simulink model "sampleModel84"  (Simulink 9.1)
settings: Solver=VariableStepAuto  StartTime=0.0  StopTime=10.0  RelTol=1e-3
undefined symbols (not defined in the file): DiscIntNeverNeededParam, Newton, Raphson
libraries: simulink x55
(part 1 of 2)
settings Model: SuppressorTable="22 serialization::archive 11 0 6 0 0 1 8 0 0 0 0 6 0 0 1 0 21 sampleModel84/cfblk80 0 6 0 0 2 8 0 0 0 0 6 41 Simulink:DataType:WarningOverFlowDetected 0 0 0 6 0  0  0 0 0 0 8 20160523 0 0 0 10 57 55 0 1 40 SimulinkFixedPoint:util:Overflowoccurred 0 0 0  0  8 20160523 0 10 57 55 0 1"  Creator=DELL  LastModifiedBy=DELL
settings DataIOCC: SaveFormat=Dataset
settings OptimizationCC: LifeSpan=auto
settings DebuggingCC: UnderspecifiedInitializationDetection=Simplified  MergeDetectMultiDrivingBlocksExec=error  SFUnexpectedBacktrackingDiag=error  SFNoUnconditionalDefaultTransitionDiag=error  SFExecutionAtInitializationDiag=warning
settings HardwareCC: ProdBitPerPointer=64  ProdBitPerSizeT=64  ProdBitPerPtrDiffT=64  ProdLargestAtomicFloat=Float  ProdIntDivRoundTo=Zero  ProdEndianess=LittleEndian  ProdWordSize=64  ProdHWDeviceType=Intel->x86-64 (Windows64)
settings ModelReferenceCC: PropagateSignalLabelsOutOfModel=on
settings CodeAppCC: StateflowObjectComments=off
settings GRTTargetCC: TargetLangStandard=C99 (ISO)  CombineOutputUpdateFcns=on  GRTInterface=off
settings ConfigComp: CovMetricSettings=dwe  CovHtmlReporting=off  CovSaveCumulativeToWorkspaceVar=off  CovSaveSingleToWorkspaceVar=off  CovExternalEMLEnable=on

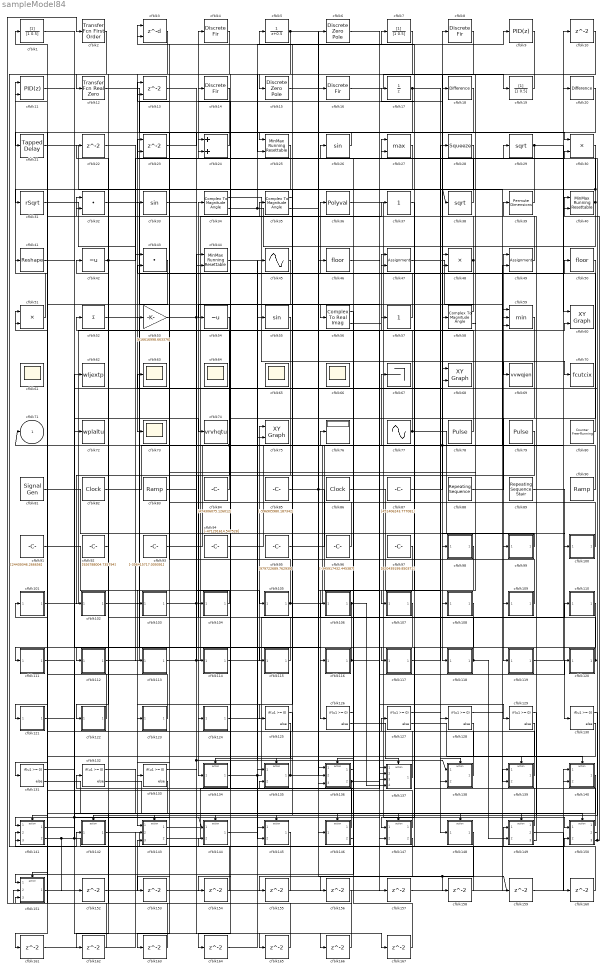
== system sampleModel84 ==
  cfblk1 : DiscreteFilter  SampleTime=1
  cfblk{10,22,152..167} (18 alike) : Delay  SampleTime=1
  cfblk100 : Subsystem
  cfblk101 : Subsystem
  cfblk102 : Subsystem
  cfblk103 : Subsystem
  cfblk104 : Subsystem
  cfblk105 : Subsystem
  cfblk106 : Subsystem
  cfblk107 : Subsystem
  cfblk108 : Subsystem
  cfblk109 : Subsystem
  cfblk11 : simulink/Continuous/PID Controller (2DOF)  Controller=PID  TimeDomain=Discrete-time  SampleTime=1  IntegratorMethod=Forward Euler  FilterMethod=Forward Euler  Form=Parallel  UseFilter=on  ControllerParametersSource=internal  P=1  I=1  D=0  N=100  b=1  c=1  InitialConditionSource=internal  InitialConditionForIntegrator=0  InitialConditionForFilter=0  ExternalReset=none  LimitOutput=off  UpperSaturationLimit=inf  LowerSaturationLimit=-inf  LinearizeAsGain=off  AntiWindupMode=none  Kb=1  TrackingMode=off  Kt=1  PParamMin=[]  PParamMax=[]  IParamMin=[]  IParamMax=[]  DParamMin=[]  DParamMax=[]  NParamMin=[]  NParamMax=[]  bParamMin=[]  bParamMax=[]  cParamMin=[]  cParamMax=[]  KbParamMin=[]  KbParamMax=[]  KtParamMin=[]  KtParamMax=[]  POutMin=[]  POutMax=[]  IOutMin=[]  IOutMax=[]  DOutMin=[]  DOutMax=[]  NOutMin=[]  NOutMax=[]  bOutMin=[]  bOutMax=[]  cOutMin=[]  cOutMax=[]  KbOutMin=[]  KbOutMax=[]  KtOutMin=[]  KtOutMax=[]  IntegratorOutMin=[]  IntegratorOutMax=[]  FilterOutMin=[]  FilterOutMax=[]  SumOutMin=[]  SumOutMax=[]  Sum1OutMin=[]  Sum1OutMax=[]  Sum2OutMin=[]  Sum2OutMax=[]  Sum3OutMin=[]  Sum3OutMax=[]  SumI1OutMin=[]  SumI1OutMax=[]  SumI2OutMin=[]  SumI2OutMax=[]  SumI3OutMin=[]  SumI3OutMax=[]  SumDOutMin=[]  SumDOutMax=[]  SaturationOutMin=[]  SaturationOutMax=[]  IntegratorContinuousStateAttributes=''  IntegratorStateMustResolveToSignalObject=off  IntegratorRTWStateStorageClass=Auto  FilterContinuousStateAttributes=''  FilterStateMustResolveToSignalObject=off  FilterRTWStateStorageClass=Auto  DifferentiatorICPrevScaledInput=0  DifferentiatorOutMin=[]  DifferentiatorOutMax=[]  FilterDiffOutCoefMin=[]  FilterDiffOutCoefMax=[]  SumDenOutMin=[]  SumDenOutMax=[]  SumNumOutMin=[]  SumNumOutMax=[]  ReciprocalOutMin=[]  ReciprocalOutMax=[]  DivideOutMin=[]  DivideOutMax=[]  TunerSelectOption=Transfer Function Based (PID Tuner App)
  cfblk110 : Subsystem
  cfblk111 : Subsystem
  cfblk112 : Subsystem
  cfblk113 : Subsystem
  cfblk114 : Subsystem
  cfblk115 : Subsystem
  cfblk116 : Subsystem
  cfblk117 : Subsystem
  cfblk118 : Subsystem
  cfblk119 : Subsystem
  cfblk12 : simulink/Discrete/Transfer Fcn Real Zero  ZeroZ=0.75  ICPrevInput=0.0  DoSatur=off
      settings: SourceProductName=Simulink  SourceProductBaseCode=SL
  cfblk120 : Subsystem
  cfblk121 : Subsystem
  cfblk122 : Subsystem
  cfblk123 : Subsystem
  cfblk124 : Subsystem
  cfblk{125..133} (9 alike) : If  IfExpression=u1 >= 0  SampleTime=1
  cfblk13 : Delay  ShowEnablePort=on  SampleTime=1
      settings: InputPortMap=u0,e6
  cfblk134 : Subsystem  TreatAsAtomicUnit=on
  cfblk135 : Subsystem  TreatAsAtomicUnit=on
  cfblk136 : Subsystem  TreatAsAtomicUnit=on
  cfblk137 : Subsystem  TreatAsAtomicUnit=on
  cfblk138 : Subsystem  TreatAsAtomicUnit=on
  cfblk139 : Subsystem  TreatAsAtomicUnit=on
  cfblk{4,8,14,16} (4 alike) : DiscreteFir  SampleTime=1
  cfblk140 : Subsystem  TreatAsAtomicUnit=on
  cfblk141 : Subsystem  TreatAsAtomicUnit=on
  cfblk142 : Subsystem  TreatAsAtomicUnit=on
  cfblk143 : Subsystem  TreatAsAtomicUnit=on
  cfblk144 : Subsystem  TreatAsAtomicUnit=on
  cfblk145 : Subsystem  TreatAsAtomicUnit=on
  cfblk146 : Subsystem  TreatAsAtomicUnit=on
  cfblk147 : Subsystem  TreatAsAtomicUnit=on
  cfblk148 : Subsystem  TreatAsAtomicUnit=on
  cfblk149 : Subsystem  TreatAsAtomicUnit=on
  cfblk15 : DiscreteZeroPole  Poles=[0 0.5]  Gain=1
  cfblk150 : Subsystem  TreatAsAtomicUnit=on
  cfblk151 : Subsystem  TreatAsAtomicUnit=on
  cfblk17 : UnitDelay
  cfblk18 : simulink/Discrete/Difference  ICPrevInput=0.0  OutMin=[]  OutMax=[]  OutDataTypeStr=Inherit: Inherit via back propagation  OutDataType=fixdt(1, 16)  OutScaling=2^-10  DoSatur=off
  cfblk19 : DiscreteFilter  SampleTime=1
  cfblk2 : simulink/Discrete/Transfer Fcn First Order  PoleZ=0.95  ICPrevOutput=0.0  DoSatur=off
      settings: SourceProductName=Simulink
  cfblk20 : simulink/Discrete/Difference  ICPrevInput=0.0  OutMin=[]  OutMax=[]  OutDataTypeStr=Inherit: Inherit via back propagation  OutDataType=fixdt(1, 16)  OutScaling=2^-10  DoSatur=off
  cfblk21 : simulink/Discrete/Tapped Delay  vinit=0.0  samptime=-1  NumDelays=1  DelayOrder=Oldest  includeCurrent=off
  cfblk23 : Delay  ShowEnablePort=on  SampleTime=1
      settings: InputPortMap=u0,e6
  cfblk24 : Sum
  cfblk25 : simulink/Math Operations/MinMax Running Resettable  Function=min  vinit=0.0
  cfblk26 : Trigonometry
  cfblk27 : MinMax  Function=max  Inputs=2
  cfblk28 : Squeeze
  cfblk29 : Sqrt  SaturateOnIntegerOverflow=on
  cfblk3 : Delay  DelayLengthSource=Input port  SampleTime=1
      settings: InputPortMap=u0,p1
  cfblk30 : Product
  cfblk31 : Sqrt  Operator=rSqrt  AlgorithmType=Newton-Raphson  SaturateOnIntegerOverflow=on
  cfblk32 : DotProduct  InputSameDT=on  OutDataTypeStr=Inherit: Inherit via internal rule
  cfblk33 : Trigonometry
  cfblk34 : ComplexToMagnitudeAngle
  cfblk35 : ComplexToMagnitudeAngle
  cfblk36 : Polyval  Coefs=[ +2.081618890e-019, -1.441693666e-014, +4.719686976e-010, -8.536869453e-006, +1.621573104e-001, -8.087801117e+001 ]
  cfblk37 : simulink/Math Operations/Slider Gain  gain=1  low=0  high=2
  cfblk38 : Sqrt  SaturateOnIntegerOverflow=on
  cfblk39 : PermuteDimensions
  cfblk40 : simulink/Math Operations/MinMax Running Resettable  Function=min  vinit=0.0
  cfblk41 : Reshape
  cfblk42 : UnaryMinus
  cfblk43 : DotProduct  InputSameDT=on  OutDataTypeStr=Inherit: Inherit via internal rule
  cfblk44 : simulink/Math Operations/MinMax Running Resettable  Function=min  vinit=0.0
  cfblk45 : Sin  TimeSource=Use external signal  SampleTime=0
  cfblk46 : Rounding
  cfblk47 : Assignment  DiagnosticForDimensions=Warning  IndexOptions=Index vector (dialog)  Indices=1  OutputSizes=1
  cfblk48 : Product  Inputs=**
  cfblk49 : Assignment  DiagnosticForDimensions=Warning  IndexOptions=Index vector (dialog)  Indices=1  OutputSizes=1
  cfblk5 : DiscreteTransferFcn  SampleTime=1
  cfblk50 : Rounding
  cfblk51 : Product  Inputs=**
  cfblk52 : Sum  Inputs=+
  cfblk53 : Gain  Gain=[616616998.663376]
  cfblk54 : UnaryMinus
  cfblk55 : Trigonometry
  cfblk56 : ComplexToRealImag
  cfblk57 : simulink/Math Operations/Slider Gain  gain=1  low=0  high=2
  cfblk58 : ComplexToMagnitudeAngle
  cfblk59 : MinMax  Inputs=3
  cfblk6 : DiscreteZeroPole  Poles=[0 0.5]  Gain=1
  cfblk60 : simulink/Sinks/XY Graph  xmin=-1  xmax=1  ymin=-1  ymax=1  st=-1
  cfblk{61,63..66,73} (6 alike) : Scope
      cfblk61 settings: Floating=on
      cfblk64 settings: Floating=on
      cfblk65 settings: Floating=on
      cfblk66 settings: Floating=on
  cfblk62 : ToWorkspace  VariableName=wljextp  SaveFormat=Timeseries  SampleTime=-1
  cfblk67 : Terminator
  cfblk68 : simulink/Sinks/XY Graph  xmin=-1  xmax=1  ymin=-1  ymax=1  st=-1
  cfblk69 : ToWorkspace  VariableName=vvwqjen  SaveFormat=Timeseries  SampleTime=-1
  cfblk7 : DiscreteFilter  SampleTime=1
  cfblk70 : ToWorkspace  VariableName=fcutcix  SaveFormat=Timeseries  SampleTime=-1
  cfblk72 : ToWorkspace  VariableName=wplaltu  SaveFormat=Timeseries  SampleTime=-1
  cfblk74 : ToWorkspace  VariableName=vrvhqtu  SaveFormat=Timeseries  SampleTime=-1
  cfblk75 : simulink/Sinks/XY Graph  xmin=-1  xmax=1  ymin=-1  ymax=1  st=-1
  cfblk76 : Display
  cfblk77 : Sin  Amplitude=[108722307.929304]  Bias=[-485802792.606317]  SampleTime=0
  cfblk78 : DiscretePulseGenerator  PulseType=Time based  Amplitude=[385040075.509657]  Period=[73350272.641050]  PulseWidth=5  PhaseDelay=[8.000000]
  cfblk79 : DiscretePulseGenerator  PulseType=Time based  Amplitude=[-502906939.049966]  Period=[87047927.574360]  PulseWidth=5  PhaseDelay=[5.000000]
  cfblk80 : simulink/Sources/Counter Free-Running  NumBits=[10.000000]  tsamp=-1
  cfblk81 : SignalGenerator  WaveForm=sawtooth  Amplitude=[-168191478.001369]  Units=rad/sec
  cfblk82 : DigitalClock
  cfblk83 : simulink/Sources/Ramp  slope=[-4630.726628]  start=[27.607635]  InitialOutput=[-903636.017661]
  cfblk84 : Constant  Value=[474306075.126012]  SampleTime=1
  cfblk85 : Constant  Value=[-596905980.187342]  SampleTime=1
  cfblk86 : DigitalClock
  cfblk87 : Constant  Value=[451406243.777081]  SampleTime=1
  cfblk88 : simulink/Sources/Repeating Sequence  rep_seq_t=[0 2]  rep_seq_y=[-211485447.920603, -631862851.400654]
  cfblk89 : simulink/Sources/Repeating Sequence Stair  OutValues=[504633055.748347, -907869422.671242]  tsamp=-1  OutMin=[]  OutMax=[]  OutDataTypeStr=double  OutputDataTypeScalingMode=double  OutDataType=fixdt(0,8)  ConRadixGroup=Best Precision: Vector-wise  OutScaling=2^-12
  cfblk9 : simulink/Continuous/PID Controller  Controller=PID  TimeDomain=Discrete-time  SampleTime=1  IntegratorMethod=Forward Euler  FilterMethod=Forward Euler  Form=Parallel  UseFilter=on  ControllerParametersSource=internal  P=1  I=1  D=0  N=100  InitialConditionSource=internal  InitialConditionForIntegrator=0  InitialConditionForFilter=0  ExternalReset=none  LimitOutput=off  UpperSaturationLimit=inf  LowerSaturationLimit=-inf  LinearizeAsGain=off  AntiWindupMode=none  Kb=1  TrackingMode=off  Kt=1  PParamMin=[]  PParamMax=[]  IParamMin=[]  IParamMax=[]  DParamMin=[]  DParamMax=[]  NParamMin=[]  NParamMax=[]  KbParamMin=[]  KbParamMax=[]  KtParamMin=[]  KtParamMax=[]  POutMin=[]  POutMax=[]  IOutMin=[]  IOutMax=[]  DOutMin=[]  DOutMax=[]  NOutMin=[]  NOutMax=[]  KbOutMin=[]  KbOutMax=[]  KtOutMin=[]  KtOutMax=[]  IntegratorOutMin=[]  IntegratorOutMax=[]  FilterOutMin=[]  FilterOutMax=[]  SumOutMin=[]  SumOutMax=[]  SumI1OutMin=[]  SumI1OutMax=[]  SumI2OutMin=[]  SumI2OutMax=[]  SumI3OutMin=[]  SumI3OutMax=[]  SumDOutMin=[]  SumDOutMax=[]  SaturationOutMin=[]  SaturationOutMax=[]  IntegratorContinuousStateAttributes=''  IntegratorStateMustResolveToSignalObject=off  IntegratorRTWStateStorageClass=Auto  FilterContinuousStateAttributes=''  FilterStateMustResolveToSignalObject=off  FilterRTWStateStorageClass=Auto  DifferentiatorICPrevScaledInput=0  DifferentiatorOutMin=[]  DifferentiatorOutMax=[]  FilterDiffOutCoefMin=[]  FilterDiffOutCoefMax=[]  SumDenOutMin=[]  SumDenOutMax=[]  SumNumOutMin=[]  SumNumOutMax=[]  ReciprocalOutMin=[]  ReciprocalOutMax=[]  DivideOutMin=[]  DivideOutMax=[]  TunerSelectOption=Transfer Function Based (PID Tuner App)
  cfblk90 : simulink/Sources/Ramp  slope=[-8360.756305]  start=[2.779328]  InitialOutput=[-108037.496599]
  cfblk91 : Constant  Value=[24439346.266656]  SampleTime=1
  cfblk92 : Constant  Value=[926788004.735794]  SampleTime=1
  cfblk93 : Constant  Value=[-356415717.009391]  SampleTime=1
  cfblk94 : Constant  Value=[-471291614.547528]  SampleTime=1
  cfblk95 : Constant  Value=[979722689.762939]  SampleTime=1
  cfblk96 : Constant  Value=[-345917432.445387]  SampleTime=1
  cfblk97 : Constant  Value=[820439199.850371]  SampleTime=1
  cfblk98 : Subsystem
  cfblk99 : Subsystem
  cfblk71 : Outport
  wires:
  cfblk82/1 -> cfblk8/1
  cfblk79/1 -> cfblk134/1(cfblk1)
  cfblk57/1 -> cfblk36/1
  cfblk97/1 -> cfblk126/1
  cfblk9/1 -> cfblk141/1(cfblk1)
  cfblk116/1(cfblk2) -> cfblk111/1(cfblk1), cfblk129/1
  cfblk52/1 -> cfblk116/1(cfblk1)
  cfblk2/1 -> cfblk142/1(cfblk1)
  cfblk89/1 -> cfblk130/1
  cfblk56/1 -> cfblk151/1(cfblk1)
  cfblk91/1 -> cfblk143/1(cfblk1)
  cfblk51/1 -> cfblk11/1
  cfblk84/1 -> cfblk71/1, cfblk13/2
  cfblk36/1 -> cfblk150/1(cfblk1)
  cfblk106/1(cfblk2) -> cfblk121/1(cfblk1), cfblk137/4(cfblk9)
  cfblk102/1(cfblk2) -> cfblk50/1
  cfblk8/1 -> cfblk118/1(cfblk1)
  cfblk93/1 -> cfblk48/1
  cfblk87/1 -> cfblk58/1
  cfblk137/1(cfblk2) -> cfblk26/1
  cfblk101/1(cfblk2) -> cfblk47/1
  cfblk113/1(cfblk2) -> cfblk37/1, cfblk48/2
  cfblk3/1 -> cfblk112/1(cfblk1)
  cfblk81/1 -> cfblk100/1(cfblk1)
  cfblk59/1 -> cfblk119/1(cfblk1)
  cfblk77/1 -> cfblk109/1(cfblk1), cfblk32/2
  cfblk37/1 -> cfblk107/1(cfblk1)
  cfblk5/1 -> cfblk158/1, cfblk159/1, cfblk25/2
  cfblk56/2 -> cfblk57/1
  cfblk112/1(cfblk2) -> cfblk18/1
  cfblk34/1 -> cfblk70/1
  cfblk119/1(cfblk2) -> cfblk20/1
  cfblk90/1 -> cfblk42/1, cfblk68/1
  cfblk35/1 -> cfblk123/1(cfblk1)
  cfblk40/1 -> cfblk38/1, cfblk13/1, cfblk138/2(cfblk11)
  cfblk136/1(cfblk2) -> cfblk76/1
  cfblk95/1 -> cfblk67/1
  cfblk118/1(cfblk2) -> cfblk34/1, cfblk149/2(cfblk13)
  cfblk7/1 -> cfblk54/1
  cfblk10/1 -> cfblk12/1
  cfblk14/1 -> cfblk73/1
  cfblk142/1(cfblk2) -> cfblk150/2(cfblk8)
  cfblk88/1 -> cfblk49/1
  cfblk38/1 -> cfblk4/1
  cfblk45/1 -> cfblk114/1(cfblk1)
  cfblk17/1 -> cfblk99/1(cfblk1), cfblk163/1
  cfblk114/1(cfblk2) -> cfblk75/1
  cfblk16/1 -> cfblk19/1
  cfblk99/1(cfblk2) -> cfblk98/1(cfblk1)
  cfblk151/1(cfblk2) -> cfblk55/1
  cfblk78/1 -> cfblk24/1
  cfblk149/1(cfblk2) -> cfblk3/1
  cfblk141/1(cfblk2) -> cfblk62/1
  cfblk47/1 -> cfblk139/2(cfblk12)
  cfblk4/1 -> cfblk53/1
  cfblk1/1 -> cfblk74/1
  cfblk20/1 -> cfblk131/1
  cfblk146/1(cfblk2) -> cfblk14/1
  cfblk33/1 -> cfblk105/1(cfblk1)
  cfblk96/1 -> cfblk23/1
  cfblk28/1 -> cfblk31/1
  cfblk48/1 -> cfblk1/1, cfblk75/2
  cfblk32/1 -> cfblk137/1(cfblk1)
  cfblk134/1(cfblk2) -> cfblk6/1, cfblk147/2(cfblk6)
  cfblk109/1(cfblk2) -> cfblk35/1
  cfblk124/1(cfblk2) -> cfblk16/1
  cfblk139/1(cfblk2) -> cfblk24/2
  cfblk100/1(cfblk2) -> cfblk23/2
  cfblk22/1 -> cfblk43/1
  cfblk108/1(cfblk2) -> cfblk117/1(cfblk1)
  cfblk86/1 -> cfblk128/1
  cfblk12/1 -> cfblk146/1(cfblk1)
  cfblk145/1(cfblk2) -> cfblk141/2(cfblk15)
  cfblk115/1(cfblk2) -> cfblk32/1
  cfblk31/1 -> cfblk113/1(cfblk1)
  cfblk85/1 -> cfblk136/1(cfblk1), cfblk137/3(cfblk8)
  cfblk35/2 -> cfblk27/1
  cfblk53/1 -> cfblk138/1(cfblk1), cfblk165/1, cfblk47/2
  cfblk42/1 -> cfblk122/1(cfblk1), cfblk30/2
  cfblk54/1 -> cfblk104/1(cfblk1)
  cfblk80/1 -> cfblk3/2
  cfblk39/1 -> cfblk33/1
  cfblk107/1(cfblk2) -> cfblk133/1
  cfblk11/1 -> cfblk115/1(cfblk1)
  cfblk120/1(cfblk2) -> cfblk27/2, cfblk40/2
  cfblk30/1 -> cfblk125/1
  cfblk150/1(cfblk2) -> cfblk7/1
  cfblk135/1(cfblk2) -> cfblk110/1(cfblk1), cfblk101/1(cfblk1)
  cfblk26/1 -> cfblk25/1
  cfblk58/1 -> cfblk56/1
  cfblk24/1 -> cfblk21/1
  cfblk150/2(cfblk9) -> cfblk63/1
  cfblk83/1 -> cfblk44/1
  cfblk21/1 -> cfblk59/1
  cfblk92/1 -> cfblk22/1
  cfblk143/1(cfblk2) -> cfblk135/2(cfblk10)
  cfblk123/1(cfblk2) -> cfblk51/1
  cfblk18/1 -> cfblk124/1(cfblk1)
  cfblk144/1(cfblk2) -> cfblk45/1
  cfblk141/2(cfblk17) -> cfblk149/1(cfblk1), cfblk68/2, cfblk152/1
  cfblk13/1 -> cfblk137/2(cfblk7)
  cfblk41/1 -> cfblk72/1
  cfblk149/3(cfblk15) -> cfblk39/1
  cfblk29/1 -> cfblk60/1, cfblk59/3
  cfblk55/1 -> cfblk102/1(cfblk1)
  cfblk105/1(cfblk2) -> cfblk43/2, cfblk49/2
  cfblk44/1 -> cfblk136/2(cfblk11)
  cfblk150/3(cfblk10) -> cfblk40/1, cfblk29/1
  cfblk103/1(cfblk2) -> cfblk145/2(cfblk10), cfblk59/2
  cfblk6/1 -> cfblk69/1
  cfblk94/1 -> cfblk10/1
  cfblk146/2(cfblk16) -> cfblk132/1
  cfblk19/1 -> cfblk15/1
  cfblk143/2(cfblk17) -> cfblk120/1(cfblk1)
  cfblk122/1(cfblk2) -> cfblk41/1
  cfblk34/2 -> cfblk148/1(cfblk1), cfblk9/1
  cfblk110/1(cfblk2) -> cfblk147/1(cfblk1)
  cfblk117/1(cfblk2) -> cfblk28/1
  cfblk58/2 -> cfblk108/1(cfblk1)
  cfblk98/1(cfblk2) -> cfblk136/3(cfblk12)
  cfblk27/1 -> cfblk44/2
  cfblk121/1(cfblk2) -> cfblk144/1(cfblk1), cfblk167/1
  cfblk147/1(cfblk2) -> cfblk51/2
  cfblk49/1 -> cfblk17/1
  cfblk23/1 -> cfblk30/1
  cfblk15/1 -> cfblk46/1
  cfblk104/1(cfblk2) -> cfblk103/1(cfblk1)
  cfblk136/2(cfblk13) -> cfblk60/2, cfblk162/1
  cfblk138/1(cfblk2) -> cfblk5/1
  cfblk125/1 -> cfblk134/Action
  cfblk125/2 -> cfblk135/Action
  cfblk126/1 -> cfblk136/Action
  cfblk126/2 -> cfblk137/Action
  cfblk127/1 -> cfblk138/Action
  cfblk127/2 -> cfblk139/Action
  cfblk128/1 -> cfblk140/Action
  cfblk128/2 -> cfblk141/Action
  cfblk129/1 -> cfblk142/Action
  cfblk129/2 -> cfblk143/Action
  cfblk130/1 -> cfblk144/Action
  cfblk130/2 -> cfblk145/Action
  cfblk131/1 -> cfblk146/Action
  cfblk131/2 -> cfblk147/Action
  cfblk132/1 -> cfblk148/Action
  cfblk132/2 -> cfblk149/Action
  cfblk133/1 -> cfblk150/Action
  cfblk133/2 -> cfblk151/Action
  cfblk152/1 -> cfblk143/3(cfblk16)
  cfblk25/1 -> cfblk153/1
  cfblk153/1 -> cfblk140/1(cfblk1)
  cfblk140/1(cfblk2) -> cfblk154/1
  cfblk154/1 -> cfblk11/2
  cfblk147/2(cfblk7) -> cfblk155/1
  cfblk155/1 -> cfblk144/2(cfblk17)
  cfblk148/1(cfblk2) -> cfblk156/1
  cfblk156/1 -> cfblk2/1
  cfblk46/1 -> cfblk157/1
  cfblk157/1 -> cfblk139/1(cfblk1)
  cfblk158/1 -> cfblk145/1(cfblk1)
  cfblk159/1 -> cfblk140/2(cfblk15)
  cfblk149/2(cfblk14) -> cfblk160/1
  cfblk160/1 -> cfblk127/1
  cfblk43/1 -> cfblk161/1
  cfblk161/1 -> cfblk143/2(cfblk15)
  cfblk162/1 -> cfblk141/3(cfblk16)
  cfblk163/1 -> cfblk151/2(cfblk8)
  cfblk50/1 -> cfblk164/1
  cfblk164/1 -> cfblk135/1(cfblk1)
  cfblk165/1 -> cfblk151/3(cfblk9)
  cfblk111/1(cfblk2) -> cfblk166/1
  cfblk166/1 -> cfblk52/1
  cfblk167/1 -> cfblk106/1(cfblk1)

== system sampleModel84/cfblk100 ==
  cfblk1 : Inport
  cfblk2 : Outport
  wires:
  cfblk1/1 -> cfblk2/1

== system sampleModel84/cfblk101 ==
  cfblk1 : Inport
  cfblk2 : Outport
  wires:
  cfblk1/1 -> cfblk2/1

== system sampleModel84/cfblk102 ==
  cfblk1 : Inport
  cfblk2 : Outport
  wires:
  cfblk1/1 -> cfblk2/1

== system sampleModel84/cfblk103 ==
  cfblk1 : Inport
  cfblk2 : Outport
  wires:
  cfblk1/1 -> cfblk2/1

== system sampleModel84/cfblk104 ==
  cfblk1 : Inport
  cfblk2 : Outport
  wires:
  cfblk1/1 -> cfblk2/1

== system sampleModel84/cfblk105 ==
  cfblk1 : Inport
  cfblk2 : Outport
  wires:
  cfblk1/1 -> cfblk2/1

== system sampleModel84/cfblk106 ==
  cfblk1 : Inport
  cfblk2 : Outport
  wires:
  cfblk1/1 -> cfblk2/1

== system sampleModel84/cfblk107 ==
  cfblk1 : Inport
  cfblk2 : Outport
  wires:
  cfblk1/1 -> cfblk2/1

== system sampleModel84/cfblk108 ==
  cfblk1 : Inport
  cfblk2 : Outport
  wires:
  cfblk1/1 -> cfblk2/1

== system sampleModel84/cfblk109 ==
  cfblk1 : Inport
  cfblk2 : Outport
  wires:
  cfblk1/1 -> cfblk2/1

== system sampleModel84/cfblk110 ==
  cfblk1 : Inport
  cfblk2 : Outport
  wires:
  cfblk1/1 -> cfblk2/1

== system sampleModel84/cfblk111 ==
  cfblk1 : Inport
  cfblk2 : Outport
  wires:
  cfblk1/1 -> cfblk2/1

== system sampleModel84/cfblk112 ==
  cfblk1 : Inport
  cfblk2 : Outport
  wires:
  cfblk1/1 -> cfblk2/1

== system sampleModel84/cfblk113 ==
  cfblk1 : Inport
  cfblk2 : Outport
  wires:
  cfblk1/1 -> cfblk2/1

== system sampleModel84/cfblk114 ==
  cfblk1 : Inport
  cfblk2 : Outport
  wires:
  cfblk1/1 -> cfblk2/1

== system sampleModel84/cfblk115 ==
  cfblk1 : Inport
  cfblk2 : Outport
  wires:
  cfblk1/1 -> cfblk2/1

== system sampleModel84/cfblk116 ==
  cfblk1 : Inport
  cfblk2 : Outport
  wires:
  cfblk1/1 -> cfblk2/1

== system sampleModel84/cfblk117 ==
  cfblk1 : Inport
  cfblk2 : Outport
  wires:
  cfblk1/1 -> cfblk2/1

== system sampleModel84/cfblk118 ==
  cfblk1 : Inport
  cfblk2 : Outport
  wires:
  cfblk1/1 -> cfblk2/1

== system sampleModel84/cfblk119 ==
  cfblk1 : Inport
  cfblk2 : Outport
  wires:
  cfblk1/1 -> cfblk2/1

== system sampleModel84/cfblk120 ==
  cfblk1 : Inport
  cfblk2 : Outport
  wires:
  cfblk1/1 -> cfblk2/1

== system sampleModel84/cfblk121 ==
  cfblk1 : Inport
  cfblk2 : Outport
  wires:
  cfblk1/1 -> cfblk2/1

== system sampleModel84/cfblk122 ==
  cfblk1 : Inport
  cfblk2 : Outport
  wires:
  cfblk1/1 -> cfblk2/1

== system sampleModel84/cfblk123 ==
  cfblk1 : Inport
  cfblk2 : Outport
  wires:
  cfblk1/1 -> cfblk2/1

== system sampleModel84/cfblk124 ==
  cfblk1 : Inport
  cfblk2 : Outport
  wires:
  cfblk1/1 -> cfblk2/1

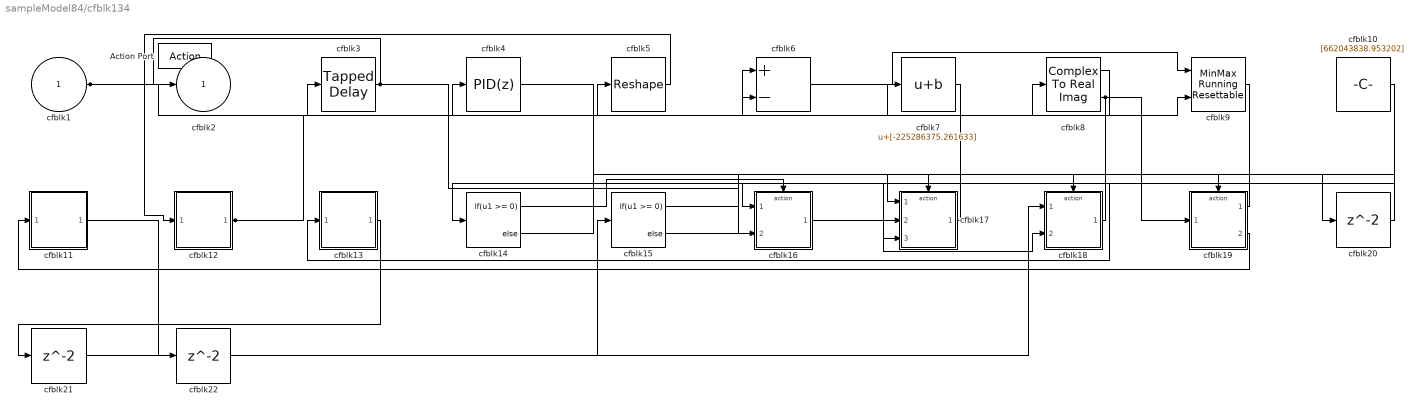
== system sampleModel84/cfblk134 ==
  cfblk1 : Inport
  Action Port : ActionPort  ActionType=then
  cfblk10 : Constant  Value=[662043838.953202]  SampleTime=1
  cfblk11 : Subsystem
  cfblk12 : Subsystem
  cfblk13 : Subsystem
  cfblk14 : If  IfExpression=u1 >= 0  SampleTime=1
  cfblk15 : If  IfExpression=u1 >= 0  SampleTime=1
  cfblk16 : Subsystem  TreatAsAtomicUnit=on
  cfblk17 : Subsystem  TreatAsAtomicUnit=on
  cfblk18 : Subsystem  TreatAsAtomicUnit=on
  cfblk19 : Subsystem  TreatAsAtomicUnit=on
  cfblk20 : Delay
  cfblk21 : Delay
  cfblk22 : Delay
  cfblk3 : simulink/Discrete/Tapped Delay  vinit=0.0  samptime=-1  NumDelays=1  DelayOrder=Oldest  includeCurrent=off
  cfblk4 : simulink/Continuous/PID Controller  Controller=PID  TimeDomain=Discrete-time  SampleTime=-1  IntegratorMethod=Forward Euler  FilterMethod=Forward Euler  Form=Parallel  UseFilter=on  ControllerParametersSource=internal  P=1  I=1  D=0  N=100  InitialConditionSource=internal  InitialConditionForIntegrator=0  InitialConditionForFilter=0  ExternalReset=none  LimitOutput=off  UpperSaturationLimit=inf  LowerSaturationLimit=-inf  LinearizeAsGain=off  AntiWindupMode=none  Kb=1  TrackingMode=off  Kt=1  PParamMin=[]  PParamMax=[]  IParamMin=[]  IParamMax=[]  DParamMin=[]  DParamMax=[]  NParamMin=[]  NParamMax=[]  KbParamMin=[]  KbParamMax=[]  KtParamMin=[]  KtParamMax=[]  POutMin=[]  POutMax=[]  IOutMin=[]  IOutMax=[]  DOutMin=[]  DOutMax=[]  NOutMin=[]  NOutMax=[]  KbOutMin=[]  KbOutMax=[]  KtOutMin=[]  KtOutMax=[]  IntegratorOutMin=[]  IntegratorOutMax=[]  FilterOutMin=[]  FilterOutMax=[]  SumOutMin=[]  SumOutMax=[]  SumI1OutMin=[]  SumI1OutMax=[]  SumI2OutMin=[]  SumI2OutMax=[]  SumI3OutMin=[]  SumI3OutMax=[]  SumDOutMin=[]  SumDOutMax=[]  SaturationOutMin=[]  SaturationOutMax=[]  IntegratorContinuousStateAttributes=''  IntegratorStateMustResolveToSignalObject=off  IntegratorRTWStateStorageClass=Auto  FilterContinuousStateAttributes=''  FilterStateMustResolveToSignalObject=off  FilterRTWStateStorageClass=Auto  DifferentiatorICPrevScaledInput=0  DifferentiatorOutMin=[]  DifferentiatorOutMax=[]  FilterDiffOutCoefMin=[]  FilterDiffOutCoefMax=[]  SumDenOutMin=[]  SumDenOutMax=[]  SumNumOutMin=[]  SumNumOutMax=[]  ReciprocalOutMin=[]  ReciprocalOutMax=[]  DivideOutMin=[]  DivideOutMax=[]  TunerSelectOption=Transfer Function Based (PID Tuner App)
  cfblk5 : Reshape
  cfblk6 : Sum  Inputs=+-
  cfblk7 : Bias  Bias=[-225286375.261633]
  cfblk8 : ComplexToRealImag
  cfblk9 : simulink/Math Operations/MinMax Running Resettable  Function=min  vinit=0.0
  cfblk2 : Outport
  wires:
  cfblk9/1 -> cfblk13/1(cfblk1)
  cfblk6/1 -> cfblk9/1
  cfblk8/1 -> cfblk3/1
  cfblk3/1 -> cfblk2/1, cfblk16/2(cfblk17)
  cfblk5/1 -> cfblk12/1(cfblk1)
  cfblk10/1 -> cfblk14/1
  cfblk8/2 -> cfblk7/1, cfblk17/3(cfblk9), cfblk19/1(cfblk1)
  cfblk19/1(cfblk2) -> cfblk17/2(cfblk8)
  cfblk16/1(cfblk2) -> cfblk18/2(cfblk17)
  cfblk7/1 -> cfblk16/1(cfblk1)
  cfblk17/1(cfblk2) -> cfblk6/1
  cfblk12/1(cfblk2) -> cfblk4/1, cfblk9/2
  cfblk1/1 -> cfblk8/1, cfblk6/2
  cfblk18/1(cfblk2) -> cfblk5/1
  cfblk19/2(cfblk11) -> cfblk11/1(cfblk1)
  cfblk14/1 -> cfblk16/Action
  cfblk14/2 -> cfblk17/Action
  cfblk15/1 -> cfblk18/Action
  cfblk15/2 -> cfblk19/Action
  cfblk4/1 -> cfblk20/1
  cfblk20/1 -> cfblk17/1(cfblk1)
  cfblk13/1(cfblk2) -> cfblk21/1
  cfblk21/1 -> cfblk18/1(cfblk1)
  cfblk11/1(cfblk2) -> cfblk22/1
  cfblk22/1 -> cfblk15/1

== system sampleModel84/cfblk135 ==
  cfblk1 : Inport
  cfblk10 : Inport  Port=2
  Action Port : ActionPort  ActionType=else
  cfblk11 : Delay
  cfblk12 : Delay
  cfblk3 : Delay  DelayLengthSource=Input port
      settings: InputPortMap=u0,p1
  cfblk4 : simulink/Discrete/Transfer Fcn First Order  PoleZ=0.95  ICPrevOutput=0.0  DoSatur=off
      settings: SourceProductName=Simulink
  cfblk5 : UnitDelay  SampleTime=-1
  cfblk6 : Gain  Gain=[-758468381.474198]
  cfblk7 : Abs
  cfblk8 : PermuteDimensions
  cfblk9 : Subsystem
  cfblk2 : Outport
  wires:
  cfblk4/1 -> cfblk9/1(cfblk1)
  cfblk7/1 -> cfblk4/1
  cfblk1/1 -> cfblk3/1
  cfblk5/1 -> cfblk2/1
  cfblk6/1 -> cfblk8/1
  cfblk10/1 -> cfblk5/1
  cfblk3/1 -> cfblk7/1
  cfblk9/1(cfblk2) -> cfblk11/1
  cfblk11/1 -> cfblk3/2
  cfblk8/1 -> cfblk12/1
  cfblk12/1 -> cfblk6/1

== system sampleModel84/cfblk136 ==
  cfblk1 : Inport
  cfblk11 : Inport  Port=2
  cfblk12 : Inport  Port=3
  Action Port : ActionPort  ActionType=then
  cfblk10 : Subsystem
  cfblk14 : Delay
  cfblk3 : Delay  ShowEnablePort=on
      settings: InputPortMap=u0,e6
  cfblk4 : simulink/Discrete/Transfer Fcn Real Zero  ZeroZ=0.75  ICPrevInput=0.0  DoSatur=off
      settings: SourceProductName=Simulink  SourceProductBaseCode=SL
  cfblk5 : simulink/Continuous/PID Controller (2DOF)  Controller=PID  TimeDomain=Discrete-time  SampleTime=-1  IntegratorMethod=Forward Euler  FilterMethod=Forward Euler  Form=Parallel  UseFilter=on  ControllerParametersSource=internal  P=1  I=1  D=0  N=100  b=1  c=1  InitialConditionSource=internal  InitialConditionForIntegrator=0  InitialConditionForFilter=0  ExternalReset=none  LimitOutput=off  UpperSaturationLimit=inf  LowerSaturationLimit=-inf  LinearizeAsGain=off  AntiWindupMode=none  Kb=1  TrackingMode=off  Kt=1  PParamMin=[]  PParamMax=[]  IParamMin=[]  IParamMax=[]  DParamMin=[]  DParamMax=[]  NParamMin=[]  NParamMax=[]  bParamMin=[]  bParamMax=[]  cParamMin=[]  cParamMax=[]  KbParamMin=[]  KbParamMax=[]  KtParamMin=[]  KtParamMax=[]  POutMin=[]  POutMax=[]  IOutMin=[]  IOutMax=[]  DOutMin=[]  DOutMax=[]  NOutMin=[]  NOutMax=[]  bOutMin=[]  bOutMax=[]  cOutMin=[]  cOutMax=[]  KbOutMin=[]  KbOutMax=[]  KtOutMin=[]  KtOutMax=[]  IntegratorOutMin=[]  IntegratorOutMax=[]  FilterOutMin=[]  FilterOutMax=[]  SumOutMin=[]  SumOutMax=[]  Sum1OutMin=[]  Sum1OutMax=[]  Sum2OutMin=[]  Sum2OutMax=[]  Sum3OutMin=[]  Sum3OutMax=[]  SumI1OutMin=[]  SumI1OutMax=[]  SumI2OutMin=[]  SumI2OutMax=[]  SumI3OutMin=[]  SumI3OutMax=[]  SumDOutMin=[]  SumDOutMax=[]  SaturationOutMin=[]  SaturationOutMax=[]  IntegratorContinuousStateAttributes=''  IntegratorStateMustResolveToSignalObject=off  IntegratorRTWStateStorageClass=Auto  FilterContinuousStateAttributes=''  FilterStateMustResolveToSignalObject=off  FilterRTWStateStorageClass=Auto  DifferentiatorICPrevScaledInput=0  DifferentiatorOutMin=[]  DifferentiatorOutMax=[]  FilterDiffOutCoefMin=[]  FilterDiffOutCoefMax=[]  SumDenOutMin=[]  SumDenOutMax=[]  SumNumOutMin=[]  SumNumOutMax=[]  ReciprocalOutMin=[]  ReciprocalOutMax=[]  DivideOutMin=[]  DivideOutMax=[]  TunerSelectOption=Transfer Function Based (PID Tuner App)
  cfblk6 : Assignment  DiagnosticForDimensions=Warning  IndexOptions=Index vector (dialog)  Indices=1  OutputSizes=1
  cfblk7 : Sqrt  SaturateOnIntegerOverflow=on
  cfblk8 : Subsystem
  cfblk9 : Subsystem
  cfblk2 : Outport
  cfblk13 : Outport  Port=2
  wires:
  cfblk12/1 -> cfblk5/1, cfblk9/1(cfblk1)
  cfblk1/1 -> cfblk8/1(cfblk1)
  cfblk9/1(cfblk2) -> cfblk7/1
  cfblk5/1 -> cfblk13/1
  cfblk8/1(cfblk2) -> cfblk6/1
  cfblk4/1 -> cfblk10/1(cfblk1), cfblk3/2
  cfblk11/1 -> cfblk2/1
  cfblk6/1 -> cfblk5/2
  cfblk3/1 -> cfblk6/2
  cfblk7/1 -> cfblk3/1
  cfblk10/1(cfblk2) -> cfblk14/1
  cfblk14/1 -> cfblk4/1

== system sampleModel84/cfblk137 ==
  cfblk1 : Inport
  cfblk7 : Inport  Port=2
  cfblk8 : Inport  Port=3
  cfblk9 : Inport  Port=4
  Action Port : ActionPort  ActionType=else
  cfblk3 : DiscreteZeroPole  Poles=[0 0.5]  Gain=1  SampleTime=-1
  cfblk4 : DiscreteIntegrator  SampleTime=-1  ICPrevOutput=DiscIntNeverNeededParam  ICPrevScaledInput=DiscIntNeverNeededParam
  cfblk5 : simulink/Discrete/Tapped Delay  vinit=0.0  samptime=-1  NumDelays=1  DelayOrder=Oldest  includeCurrent=off
  cfblk6 : Squeeze
  cfblk2 : Outport
  wires:
  cfblk3/1 -> cfblk4/1
  cfblk8/1 -> cfblk2/1
  cfblk9/1 -> cfblk5/1
  cfblk6/1 -> cfblk3/1
  cfblk7/1 -> cfblk6/1

== system sampleModel84/cfblk138 ==
  cfblk1 : Inport
  cfblk11 : Inport  Port=2
  Action Port : ActionPort  ActionType=then
  cfblk10 : Subsystem
  cfblk12 : Delay
  cfblk13 : Delay
  cfblk3 : simulink/Continuous/PID Controller  Controller=PID  TimeDomain=Discrete-time  SampleTime=-1  IntegratorMethod=Forward Euler  FilterMethod=Forward Euler  Form=Parallel  UseFilter=on  ControllerParametersSource=internal  P=1  I=1  D=0  N=100  InitialConditionSource=internal  InitialConditionForIntegrator=0  InitialConditionForFilter=0  ExternalReset=none  LimitOutput=off  UpperSaturationLimit=inf  LowerSaturationLimit=-inf  LinearizeAsGain=off  AntiWindupMode=none  Kb=1  TrackingMode=off  Kt=1  PParamMin=[]  PParamMax=[]  IParamMin=[]  IParamMax=[]  DParamMin=[]  DParamMax=[]  NParamMin=[]  NParamMax=[]  KbParamMin=[]  KbParamMax=[]  KtParamMin=[]  KtParamMax=[]  POutMin=[]  POutMax=[]  IOutMin=[]  IOutMax=[]  DOutMin=[]  DOutMax=[]  NOutMin=[]  NOutMax=[]  KbOutMin=[]  KbOutMax=[]  KtOutMin=[]  KtOutMax=[]  IntegratorOutMin=[]  IntegratorOutMax=[]  FilterOutMin=[]  FilterOutMax=[]  SumOutMin=[]  SumOutMax=[]  SumI1OutMin=[]  SumI1OutMax=[]  SumI2OutMin=[]  SumI2OutMax=[]  SumI3OutMin=[]  SumI3OutMax=[]  SumDOutMin=[]  SumDOutMax=[]  SaturationOutMin=[]  SaturationOutMax=[]  IntegratorContinuousStateAttributes=''  IntegratorStateMustResolveToSignalObject=off  IntegratorRTWStateStorageClass=Auto  FilterContinuousStateAttributes=''  FilterStateMustResolveToSignalObject=off  FilterRTWStateStorageClass=Auto  DifferentiatorICPrevScaledInput=0  DifferentiatorOutMin=[]  DifferentiatorOutMax=[]  FilterDiffOutCoefMin=[]  FilterDiffOutCoefMax=[]  SumDenOutMin=[]  SumDenOutMax=[]  SumNumOutMin=[]  SumNumOutMax=[]  ReciprocalOutMin=[]  ReciprocalOutMax=[]  DivideOutMin=[]  DivideOutMax=[]  TunerSelectOption=Transfer Function Based (PID Tuner App)
  cfblk4 : DiscreteZeroPole  Poles=[0 0.5]  Gain=1  SampleTime=-1
  cfblk5 : Rounding
  cfblk6 : simulink/Math Operations/Slider Gain  gain=1  low=0  high=2
  cfblk7 : Sum  Inputs=|++
  cfblk8 : Subsystem
  cfblk9 : Subsystem
  cfblk2 : Outport
  wires:
  cfblk7/1 -> cfblk6/1
  cfblk9/1(cfblk2) -> cfblk10/1(cfblk1)
  cfblk1/1 -> cfblk3/1
  cfblk3/1 -> cfblk7/1
  cfblk11/1 -> cfblk2/1
  cfblk4/1 -> cfblk8/1(cfblk1)
  cfblk5/1 -> cfblk4/1
  cfblk6/1 -> cfblk5/1
  cfblk8/1(cfblk2) -> cfblk12/1
  cfblk12/1 -> cfblk7/2
  cfblk10/1(cfblk2) -> cfblk13/1
  cfblk13/1 -> cfblk9/1(cfblk1)

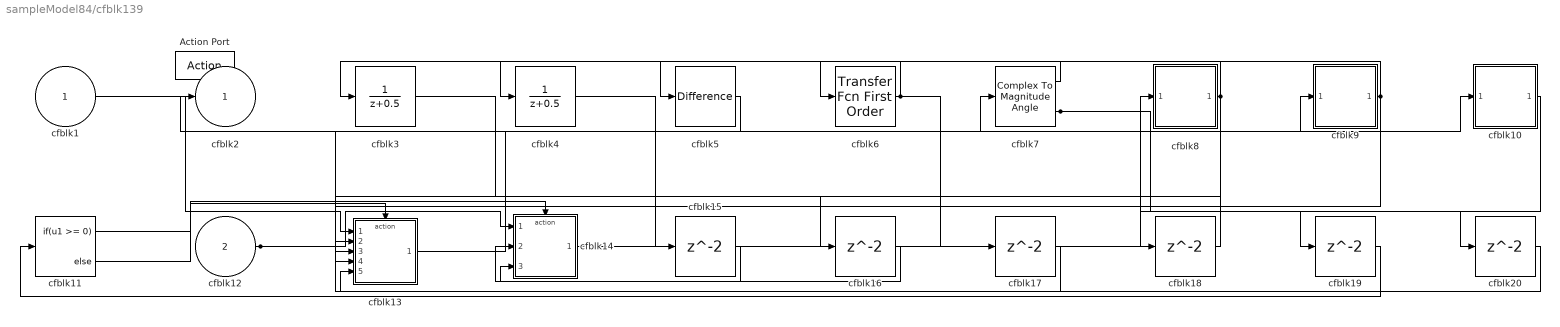
== system sampleModel84/cfblk139 ==
  cfblk1 : Inport
  cfblk12 : Inport  Port=2
  Action Port : ActionPort  ActionType=else
  cfblk10 : Subsystem
  cfblk11 : If  IfExpression=u1 >= 0  SampleTime=1
  cfblk13 : Subsystem  TreatAsAtomicUnit=on
  cfblk14 : Subsystem  TreatAsAtomicUnit=on
  cfblk{15..20} (6 alike) : Delay
  cfblk3 : DiscreteTransferFcn
  cfblk4 : DiscreteTransferFcn
  cfblk5 : simulink/Discrete/Difference  ICPrevInput=0.0  OutMin=[]  OutMax=[]  OutDataTypeStr=Inherit: Inherit via back propagation  OutDataType=fixdt(1, 16)  OutScaling=2^-10  DoSatur=off
  cfblk6 : simulink/Discrete/Transfer Fcn First Order  PoleZ=0.95  ICPrevOutput=0.0  DoSatur=off
      settings: SourceProductName=Simulink
  cfblk7 : ComplexToMagnitudeAngle
  cfblk8 : Subsystem
  cfblk9 : Subsystem
  cfblk2 : Outport
  wires:
  cfblk13/1(cfblk2) -> cfblk7/1
  cfblk12/1 -> cfblk14/1(cfblk1), cfblk9/1(cfblk1)
  cfblk7/1 -> cfblk4/1
  cfblk14/1(cfblk2) -> cfblk8/1(cfblk1)
  cfblk7/2 -> cfblk10/1(cfblk1), cfblk20/1
  cfblk9/1(cfblk2) -> cfblk5/1, cfblk13/4(cfblk13)
  cfblk6/1 -> cfblk3/1, cfblk17/1
  cfblk1/1 -> cfblk13/1(cfblk1)
  cfblk5/1 -> cfblk2/1
  cfblk8/1(cfblk2) -> cfblk6/1, cfblk18/1
  cfblk11/1 -> cfblk13/Action
  cfblk11/2 -> cfblk14/Action
  cfblk4/1 -> cfblk15/1
  cfblk15/1 -> cfblk14/2(cfblk11)
  cfblk3/1 -> cfblk16/1
  cfblk16/1 -> cfblk14/3(cfblk12)
  cfblk17/1 -> cfblk13/3(cfblk12)
  cfblk18/1 -> cfblk13/2(cfblk11)
  cfblk10/1(cfblk2) -> cfblk19/1
  cfblk19/1 -> cfblk11/1
  cfblk20/1 -> cfblk13/5(cfblk14)

== system sampleModel84/cfblk140 ==
  cfblk1 : Inport
  cfblk15 : Inport  Port=2
  Action Port : ActionPort  ActionType=then
  cfblk10 : Constant  Value=[760084940.409200]  SampleTime=1
  cfblk11 : Subsystem
  cfblk12 : Subsystem
  cfblk13 : Subsystem
  cfblk14 : Subsystem
  cfblk3 : Delay
  cfblk4 : DiscreteTransferFcn
  cfblk5 : DiscreteZeroPole  Poles=[0 0.5]  Gain=1  SampleTime=-1
  cfblk6 : DiscreteTransferFcn
  cfblk7 : DotProduct  InputSameDT=on  OutDataTypeStr=Inherit: Inherit via internal rule
  cfblk8 : Math  Operator=log10  SaturateOnIntegerOverflow=on
  cfblk9 : MinMax  Inputs=3
  cfblk2 : Outport
  wires:
  cfblk9/1 -> cfblk2/1
  cfblk4/1 -> cfblk9/1
  cfblk10/1 -> cfblk14/1(cfblk1)
  cfblk12/1(cfblk2) -> cfblk4/1, cfblk7/2
  cfblk1/1 -> cfblk12/1(cfblk1)
  cfblk5/1 -> cfblk9/2
  cfblk11/1(cfblk2) -> cfblk7/1
  cfblk3/1 -> cfblk13/1(cfblk1)
  cfblk14/1(cfblk2) -> cfblk3/1
  cfblk13/1(cfblk2) -> cfblk11/1(cfblk1)
  cfblk15/1 -> cfblk9/3
  cfblk8/1 -> cfblk5/1
  cfblk6/1 -> cfblk8/1
  cfblk7/1 -> cfblk6/1

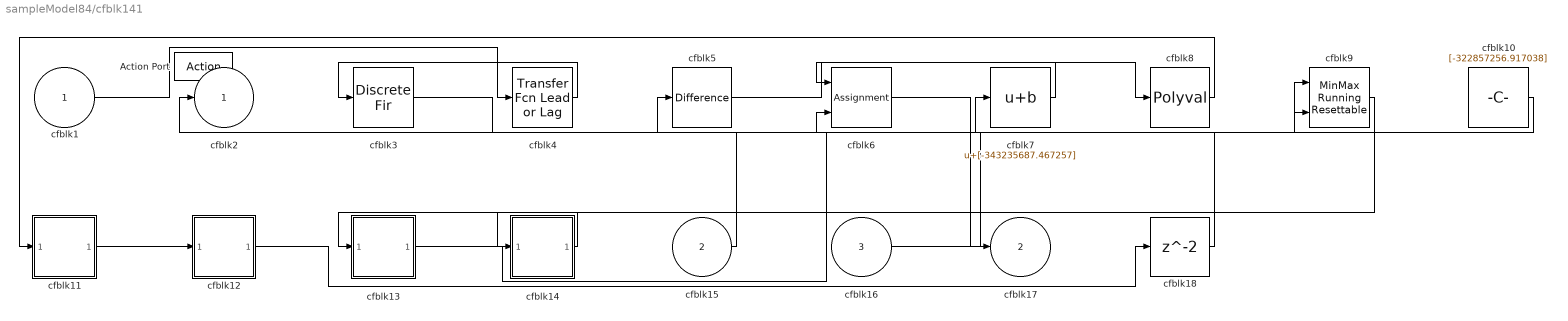
== system sampleModel84/cfblk141 ==
  cfblk1 : Inport
  cfblk15 : Inport  Port=2
  cfblk16 : Inport  Port=3
  Action Port : ActionPort  ActionType=else
  cfblk10 : Constant  Value=[-322857256.917038]  SampleTime=1
  cfblk11 : Subsystem
  cfblk12 : Subsystem
  cfblk13 : Subsystem
  cfblk14 : Subsystem
  cfblk18 : Delay
  cfblk3 : DiscreteFir
  cfblk4 : simulink/Discrete/Transfer Fcn Lead or Lag  PoleZ=0.95  ZeroZ=0.75  ICPrevOutput=0.0  ICPrevInput=0.0  DoSatur=off
      settings: SourceProductName=Simulink  SourceProductBaseCode=SL
  cfblk5 : simulink/Discrete/Difference  ICPrevInput=0.0  OutMin=[]  OutMax=[]  OutDataTypeStr=Inherit: Inherit via back propagation  OutDataType=fixdt(1, 16)  OutScaling=2^-10  DoSatur=off
  cfblk6 : Assignment  DiagnosticForDimensions=Warning  IndexOptions=Index vector (dialog)  Indices=1  OutputSizes=1
  cfblk7 : Bias  Bias=[-343235687.467257]
  cfblk8 : Polyval  Coefs=[ +2.081618890e-019, -1.441693666e-014, +4.719686976e-010, -8.536869453e-006, +1.621573104e-001, -8.087801117e+001 ]
  cfblk9 : simulink/Math Operations/MinMax Running Resettable  Function=min  vinit=0.0
  cfblk2 : Outport
  cfblk17 : Outport  Port=2
  wires:
  cfblk16/1 -> cfblk9/1
  cfblk15/1 -> cfblk2/1
  cfblk13/1(cfblk2) -> cfblk7/1
  cfblk1/1 -> cfblk4/1
  cfblk8/1 -> cfblk11/1(cfblk1)
  cfblk10/1 -> cfblk9/2
  cfblk5/1 -> cfblk8/1
  cfblk7/1 -> cfblk6/1
  cfblk4/1 -> cfblk3/1
  cfblk11/1(cfblk2) -> cfblk12/1(cfblk1)
  cfblk6/1 -> cfblk17/1
  cfblk14/1(cfblk2) -> cfblk13/1(cfblk1)
  cfblk3/1 -> cfblk6/2
  cfblk9/1 -> cfblk14/1(cfblk1)
  cfblk12/1(cfblk2) -> cfblk18/1
  cfblk18/1 -> cfblk5/1

== system sampleModel84/cfblk142 ==
  cfblk1 : Inport
  Action Port : ActionPort  ActionType=then
  cfblk3 : DiscreteFilter
  cfblk4 : simulink/Continuous/PID Controller  Controller=PID  TimeDomain=Discrete-time  SampleTime=-1  IntegratorMethod=Forward Euler  FilterMethod=Forward Euler  Form=Parallel  UseFilter=on  ControllerParametersSource=internal  P=1  I=1  D=0  N=100  InitialConditionSource=internal  InitialConditionForIntegrator=0  InitialConditionForFilter=0  ExternalReset=none  LimitOutput=off  UpperSaturationLimit=inf  LowerSaturationLimit=-inf  LinearizeAsGain=off  AntiWindupMode=none  Kb=1  TrackingMode=off  Kt=1  PParamMin=[]  PParamMax=[]  IParamMin=[]  IParamMax=[]  DParamMin=[]  DParamMax=[]  NParamMin=[]  NParamMax=[]  KbParamMin=[]  KbParamMax=[]  KtParamMin=[]  KtParamMax=[]  POutMin=[]  POutMax=[]  IOutMin=[]  IOutMax=[]  DOutMin=[]  DOutMax=[]  NOutMin=[]  NOutMax=[]  KbOutMin=[]  KbOutMax=[]  KtOutMin=[]  KtOutMax=[]  IntegratorOutMin=[]  IntegratorOutMax=[]  FilterOutMin=[]  FilterOutMax=[]  SumOutMin=[]  SumOutMax=[]  SumI1OutMin=[]  SumI1OutMax=[]  SumI2OutMin=[]  SumI2OutMax=[]  SumI3OutMin=[]  SumI3OutMax=[]  SumDOutMin=[]  SumDOutMax=[]  SaturationOutMin=[]  SaturationOutMax=[]  IntegratorContinuousStateAttributes=''  IntegratorStateMustResolveToSignalObject=off  IntegratorRTWStateStorageClass=Auto  FilterContinuousStateAttributes=''  FilterStateMustResolveToSignalObject=off  FilterRTWStateStorageClass=Auto  DifferentiatorICPrevScaledInput=0  DifferentiatorOutMin=[]  DifferentiatorOutMax=[]  FilterDiffOutCoefMin=[]  FilterDiffOutCoefMax=[]  SumDenOutMin=[]  SumDenOutMax=[]  SumNumOutMin=[]  SumNumOutMax=[]  ReciprocalOutMin=[]  ReciprocalOutMax=[]  DivideOutMin=[]  DivideOutMax=[]  TunerSelectOption=Transfer Function Based (PID Tuner App)
  cfblk5 : Subsystem
  cfblk6 : Subsystem
  cfblk7 : Subsystem
  cfblk8 : Delay
  cfblk2 : Outport
  wires:
  cfblk4/1 -> cfblk5/1(cfblk1)
  cfblk7/1(cfblk2) -> cfblk6/1(cfblk1)
  cfblk6/1(cfblk2) -> cfblk4/1
  cfblk3/1 -> cfblk7/1(cfblk1)
  cfblk1/1 -> cfblk2/1
  cfblk5/1(cfblk2) -> cfblk8/1
  cfblk8/1 -> cfblk3/1

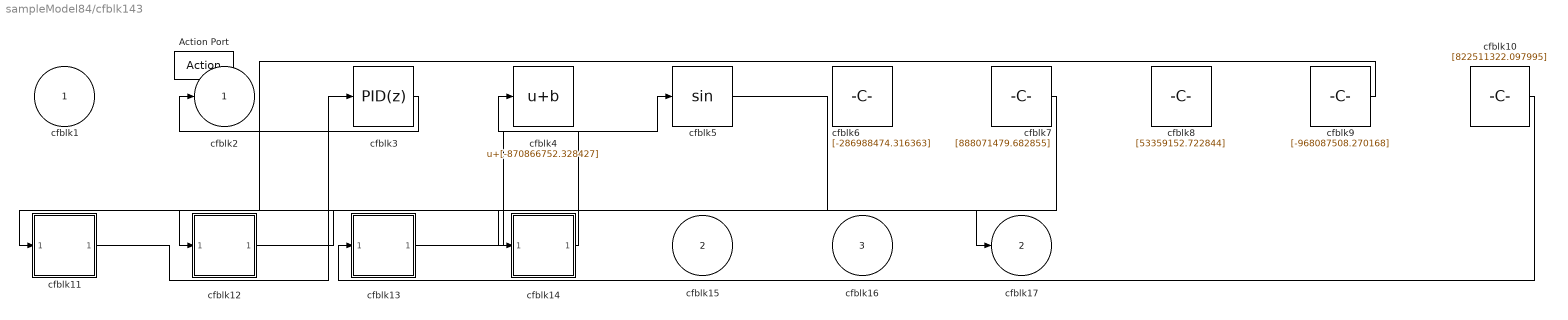
== system sampleModel84/cfblk143 ==
  cfblk1 : Inport
  cfblk15 : Inport  Port=2
  cfblk16 : Inport  Port=3
  Action Port : ActionPort  ActionType=else
  cfblk10 : Constant  Value=[822511322.097995]  SampleTime=1
  cfblk11 : Subsystem
  cfblk12 : Subsystem
  cfblk13 : Subsystem
  cfblk14 : Subsystem
  cfblk3 : simulink/Continuous/PID Controller  Controller=PID  TimeDomain=Discrete-time  SampleTime=-1  IntegratorMethod=Forward Euler  FilterMethod=Forward Euler  Form=Parallel  UseFilter=on  ControllerParametersSource=internal  P=1  I=1  D=0  N=100  InitialConditionSource=internal  InitialConditionForIntegrator=0  InitialConditionForFilter=0  ExternalReset=none  LimitOutput=off  UpperSaturationLimit=inf  LowerSaturationLimit=-inf  LinearizeAsGain=off  AntiWindupMode=none  Kb=1  TrackingMode=off  Kt=1  PParamMin=[]  PParamMax=[]  IParamMin=[]  IParamMax=[]  DParamMin=[]  DParamMax=[]  NParamMin=[]  NParamMax=[]  KbParamMin=[]  KbParamMax=[]  KtParamMin=[]  KtParamMax=[]  POutMin=[]  POutMax=[]  IOutMin=[]  IOutMax=[]  DOutMin=[]  DOutMax=[]  NOutMin=[]  NOutMax=[]  KbOutMin=[]  KbOutMax=[]  KtOutMin=[]  KtOutMax=[]  IntegratorOutMin=[]  IntegratorOutMax=[]  FilterOutMin=[]  FilterOutMax=[]  SumOutMin=[]  SumOutMax=[]  SumI1OutMin=[]  SumI1OutMax=[]  SumI2OutMin=[]  SumI2OutMax=[]  SumI3OutMin=[]  SumI3OutMax=[]  SumDOutMin=[]  SumDOutMax=[]  SaturationOutMin=[]  SaturationOutMax=[]  IntegratorContinuousStateAttributes=''  IntegratorStateMustResolveToSignalObject=off  IntegratorRTWStateStorageClass=Auto  FilterContinuousStateAttributes=''  FilterStateMustResolveToSignalObject=off  FilterRTWStateStorageClass=Auto  DifferentiatorICPrevScaledInput=0  DifferentiatorOutMin=[]  DifferentiatorOutMax=[]  FilterDiffOutCoefMin=[]  FilterDiffOutCoefMax=[]  SumDenOutMin=[]  SumDenOutMax=[]  SumNumOutMin=[]  SumNumOutMax=[]  ReciprocalOutMin=[]  ReciprocalOutMax=[]  DivideOutMin=[]  DivideOutMax=[]  TunerSelectOption=Transfer Function Based (PID Tuner App)
  cfblk4 : Bias  Bias=[-870866752.328427]
  cfblk5 : Trigonometry
  cfblk6 : Constant  Value=[-286988474.316363]  SampleTime=1
  cfblk7 : Constant  Value=[888071479.682855]  SampleTime=1
  cfblk8 : Constant  Value=[53359152.722844]  SampleTime=1
  cfblk9 : Constant  Value=[-968087508.270168]  SampleTime=1
  cfblk2 : Outport
  cfblk17 : Outport  Port=2
  wires:
  cfblk5/1 -> cfblk17/1
  cfblk9/1 -> cfblk12/1(cfblk1)
  cfblk13/1(cfblk2) -> cfblk5/1
  cfblk10/1 -> cfblk13/1(cfblk1)
  cfblk11/1(cfblk2) -> cfblk3/1
  cfblk7/1 -> cfblk11/1(cfblk1)
  cfblk12/1(cfblk2) -> cfblk14/1(cfblk1)
  cfblk3/1 -> cfblk2/1
  cfblk14/1(cfblk2) -> cfblk4/1

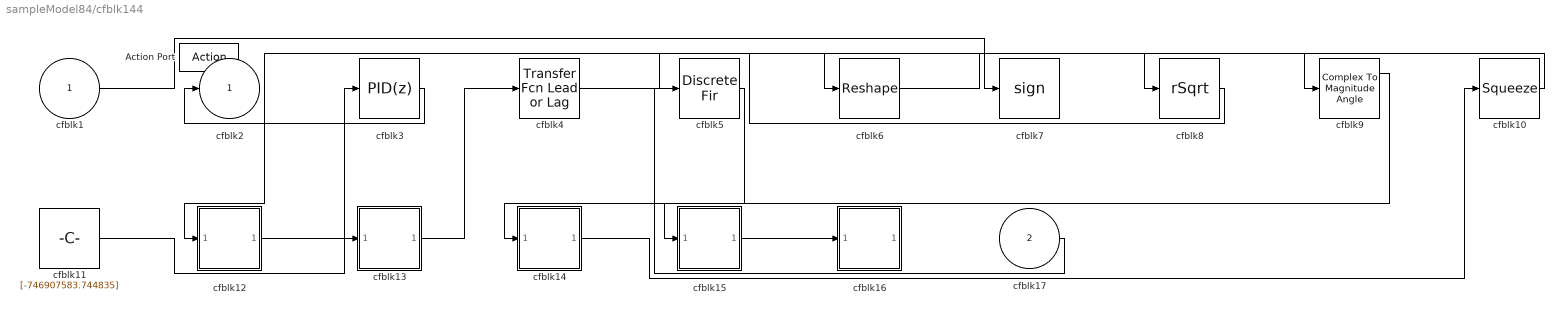
== system sampleModel84/cfblk144 ==
  cfblk1 : Inport
  cfblk17 : Inport  Port=2
  Action Port : ActionPort  ActionType=then
  cfblk10 : Squeeze
  cfblk11 : Constant  Value=[-746907583.744835]  SampleTime=1
  cfblk12 : Subsystem
  cfblk13 : Subsystem
  cfblk14 : Subsystem
  cfblk15 : Subsystem
  cfblk16 : Subsystem
  cfblk3 : simulink/Continuous/PID Controller  Controller=PID  TimeDomain=Discrete-time  SampleTime=-1  IntegratorMethod=Forward Euler  FilterMethod=Forward Euler  Form=Parallel  UseFilter=on  ControllerParametersSource=internal  P=1  I=1  D=0  N=100  InitialConditionSource=internal  InitialConditionForIntegrator=0  InitialConditionForFilter=0  ExternalReset=none  LimitOutput=off  UpperSaturationLimit=inf  LowerSaturationLimit=-inf  LinearizeAsGain=off  AntiWindupMode=none  Kb=1  TrackingMode=off  Kt=1  PParamMin=[]  PParamMax=[]  IParamMin=[]  IParamMax=[]  DParamMin=[]  DParamMax=[]  NParamMin=[]  NParamMax=[]  KbParamMin=[]  KbParamMax=[]  KtParamMin=[]  KtParamMax=[]  POutMin=[]  POutMax=[]  IOutMin=[]  IOutMax=[]  DOutMin=[]  DOutMax=[]  NOutMin=[]  NOutMax=[]  KbOutMin=[]  KbOutMax=[]  KtOutMin=[]  KtOutMax=[]  IntegratorOutMin=[]  IntegratorOutMax=[]  FilterOutMin=[]  FilterOutMax=[]  SumOutMin=[]  SumOutMax=[]  SumI1OutMin=[]  SumI1OutMax=[]  SumI2OutMin=[]  SumI2OutMax=[]  SumI3OutMin=[]  SumI3OutMax=[]  SumDOutMin=[]  SumDOutMax=[]  SaturationOutMin=[]  SaturationOutMax=[]  IntegratorContinuousStateAttributes=''  IntegratorStateMustResolveToSignalObject=off  IntegratorRTWStateStorageClass=Auto  FilterContinuousStateAttributes=''  FilterStateMustResolveToSignalObject=off  FilterRTWStateStorageClass=Auto  DifferentiatorICPrevScaledInput=0  DifferentiatorOutMin=[]  DifferentiatorOutMax=[]  FilterDiffOutCoefMin=[]  FilterDiffOutCoefMax=[]  SumDenOutMin=[]  SumDenOutMax=[]  SumNumOutMin=[]  SumNumOutMax=[]  ReciprocalOutMin=[]  ReciprocalOutMax=[]  DivideOutMin=[]  DivideOutMax=[]  TunerSelectOption=Transfer Function Based (PID Tuner App)
  cfblk4 : simulink/Discrete/Transfer Fcn Lead or Lag  PoleZ=0.95  ZeroZ=0.75  ICPrevOutput=0.0  ICPrevInput=0.0  DoSatur=off
      settings: SourceProductName=Simulink  SourceProductBaseCode=SL
  cfblk5 : DiscreteFir
  cfblk6 : Reshape
  cfblk7 : Signum
  cfblk8 : Sqrt  Operator=rSqrt  AlgorithmType=Newton-Raphson  SaturateOnIntegerOverflow=on
  cfblk9 : ComplexToMagnitudeAngle
  cfblk2 : Outport
  wires:
  cfblk15/1(cfblk2) -> cfblk16/1(cfblk1)
  cfblk9/1 -> cfblk15/1(cfblk1)
  cfblk17/1 -> cfblk5/1
  cfblk1/1 -> cfblk7/1
  cfblk8/1 -> cfblk12/1(cfblk1)
  cfblk11/1 -> cfblk3/1
  cfblk5/1 -> cfblk14/1(cfblk1)
  cfblk3/1 -> cfblk2/1
  cfblk14/1(cfblk2) -> cfblk10/1
  cfblk10/1 -> cfblk6/1
  cfblk12/1(cfblk2) -> cfblk13/1(cfblk1)
  cfblk4/1 -> cfblk9/1
  cfblk13/1(cfblk2) -> cfblk4/1
  cfblk6/1 -> cfblk8/1

== system sampleModel84/cfblk145 ==
  cfblk1 : Inport
  cfblk10 : Inport  Port=2
  Action Port : ActionPort  ActionType=else
  cfblk11 : Delay
  cfblk12 : Delay
  cfblk3 : DiscreteStateSpace  SampleTime=-1
  cfblk4 : Sum  Inputs=--
  cfblk5 : Sum
  cfblk6 : Subsystem
  cfblk7 : Subsystem
  cfblk8 : Subsystem
  cfblk9 : Subsystem
  cfblk2 : Outport
  wires:
  cfblk10/1 -> cfblk2/1
  cfblk1/1 -> cfblk6/1(cfblk1)
  cfblk8/1(cfblk2) -> cfblk9/1(cfblk1)
  cfblk4/1 -> cfblk3/1
  cfblk6/1(cfblk2) -> cfblk5/2
  cfblk9/1(cfblk2) -> cfblk4/2, cfblk12/1
  cfblk3/1 -> cfblk7/1(cfblk1)
  cfblk5/1 -> cfblk4/1
  cfblk7/1(cfblk2) -> cfblk11/1
  cfblk11/1 -> cfblk5/1
  cfblk12/1 -> cfblk8/1(cfblk1)

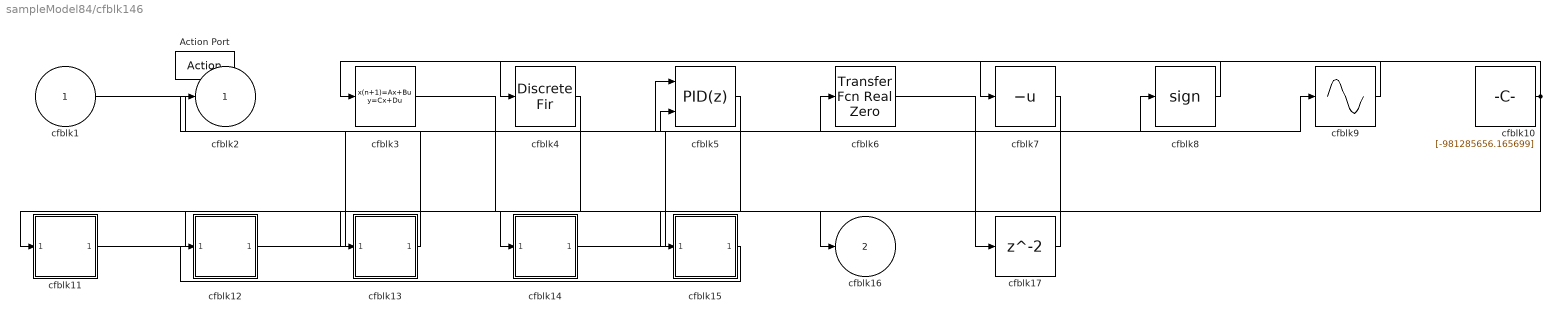
== system sampleModel84/cfblk146 ==
  cfblk1 : Inport
  Action Port : ActionPort  ActionType=then
  cfblk10 : Constant  Value=[-981285656.165699]  SampleTime=1
  cfblk11 : Subsystem
  cfblk12 : Subsystem
  cfblk13 : Subsystem
  cfblk14 : Subsystem
  cfblk15 : Subsystem
  cfblk17 : Delay
  cfblk3 : DiscreteStateSpace  SampleTime=-1
  cfblk4 : DiscreteFir
  cfblk5 : simulink/Continuous/PID Controller (2DOF)  Controller=PID  TimeDomain=Discrete-time  SampleTime=-1  IntegratorMethod=Forward Euler  FilterMethod=Forward Euler  Form=Parallel  UseFilter=on  ControllerParametersSource=internal  P=1  I=1  D=0  N=100  b=1  c=1  InitialConditionSource=internal  InitialConditionForIntegrator=0  InitialConditionForFilter=0  ExternalReset=none  LimitOutput=off  UpperSaturationLimit=inf  LowerSaturationLimit=-inf  LinearizeAsGain=off  AntiWindupMode=none  Kb=1  TrackingMode=off  Kt=1  PParamMin=[]  PParamMax=[]  IParamMin=[]  IParamMax=[]  DParamMin=[]  DParamMax=[]  NParamMin=[]  NParamMax=[]  bParamMin=[]  bParamMax=[]  cParamMin=[]  cParamMax=[]  KbParamMin=[]  KbParamMax=[]  KtParamMin=[]  KtParamMax=[]  POutMin=[]  POutMax=[]  IOutMin=[]  IOutMax=[]  DOutMin=[]  DOutMax=[]  NOutMin=[]  NOutMax=[]  bOutMin=[]  bOutMax=[]  cOutMin=[]  cOutMax=[]  KbOutMin=[]  KbOutMax=[]  KtOutMin=[]  KtOutMax=[]  IntegratorOutMin=[]  IntegratorOutMax=[]  FilterOutMin=[]  FilterOutMax=[]  SumOutMin=[]  SumOutMax=[]  Sum1OutMin=[]  Sum1OutMax=[]  Sum2OutMin=[]  Sum2OutMax=[]  Sum3OutMin=[]  Sum3OutMax=[]  SumI1OutMin=[]  SumI1OutMax=[]  SumI2OutMin=[]  SumI2OutMax=[]  SumI3OutMin=[]  SumI3OutMax=[]  SumDOutMin=[]  SumDOutMax=[]  SaturationOutMin=[]  SaturationOutMax=[]  IntegratorContinuousStateAttributes=''  IntegratorStateMustResolveToSignalObject=off  IntegratorRTWStateStorageClass=Auto  FilterContinuousStateAttributes=''  FilterStateMustResolveToSignalObject=off  FilterRTWStateStorageClass=Auto  DifferentiatorICPrevScaledInput=0  DifferentiatorOutMin=[]  DifferentiatorOutMax=[]  FilterDiffOutCoefMin=[]  FilterDiffOutCoefMax=[]  SumDenOutMin=[]  SumDenOutMax=[]  SumNumOutMin=[]  SumNumOutMax=[]  ReciprocalOutMin=[]  ReciprocalOutMax=[]  DivideOutMin=[]  DivideOutMax=[]  TunerSelectOption=Transfer Function Based (PID Tuner App)
  cfblk6 : simulink/Discrete/Transfer Fcn Real Zero  ZeroZ=0.75  ICPrevInput=0.0  DoSatur=off
      settings: SourceProductName=Simulink  SourceProductBaseCode=SL
  cfblk7 : UnaryMinus
  cfblk8 : Signum
  cfblk9 : Sin  TimeSource=Use external signal  SampleTime=0
  cfblk2 : Outport
  cfblk16 : Outport  Port=2
  wires:
  cfblk11/1(cfblk2) -> cfblk14/1(cfblk1)
  cfblk8/1 -> cfblk3/1
  cfblk1/1 -> cfblk9/1
  cfblk9/1 -> cfblk7/1
  cfblk12/1(cfblk2) -> cfblk8/1
  cfblk4/1 -> cfblk13/1(cfblk1)
  cfblk15/1(cfblk2) -> cfblk12/1(cfblk1)
  cfblk5/1 -> cfblk11/1(cfblk1)
  cfblk10/1 -> cfblk4/1, cfblk15/1(cfblk1)
  cfblk14/1(cfblk2) -> cfblk6/1
  cfblk3/1 -> cfblk16/1
  cfblk7/1 -> cfblk5/2
  cfblk13/1(cfblk2) -> cfblk2/1
  cfblk6/1 -> cfblk17/1
  cfblk17/1 -> cfblk5/1

== system sampleModel84/cfblk147 ==
  cfblk1 : Inport
  cfblk6 : Inport  Port=2
  Action Port : ActionPort  ActionType=else
  cfblk3 : simulink/Discrete/Transfer Fcn Real Zero  ZeroZ=0.75  ICPrevInput=0.0  DoSatur=off
      settings: SourceProductName=Simulink  SourceProductBaseCode=SL
  cfblk4 : Sum  Inputs=|++
  cfblk5 : Subsystem
  cfblk8 : Delay
  cfblk2 : Outport
  cfblk7 : Outport  Port=2
  wires:
  cfblk6/1 -> cfblk3/1
  cfblk5/1(cfblk2) -> cfblk2/1, cfblk8/1
  cfblk1/1 -> cfblk7/1
  cfblk3/1 -> cfblk4/2
  cfblk4/1 -> cfblk5/1(cfblk1)
  cfblk8/1 -> cfblk4/1

== system sampleModel84/cfblk148 ==
  cfblk1 : Inport
  Action Port : ActionPort  ActionType=then
  cfblk10 : Subsystem  TreatAsAtomicUnit=on
  cfblk11 : Subsystem  TreatAsAtomicUnit=on
  cfblk12 : Delay
  cfblk13 : Delay
  cfblk14 : Delay
  cfblk3 : ComplexToMagnitudeAngle
  cfblk4 : Constant  Value=[833974667.304825]  SampleTime=1
  cfblk5 : Subsystem
  cfblk6 : Subsystem
  cfblk7 : Subsystem
  cfblk8 : Subsystem
  cfblk9 : If  IfExpression=u1 >= 0  SampleTime=1
  cfblk2 : Outport
  wires:
  cfblk8/1(cfblk2) -> cfblk7/1(cfblk1)
  cfblk11/1(cfblk2) -> cfblk6/1(cfblk1)
  cfblk1/1 -> cfblk9/1
  cfblk7/1(cfblk2) -> cfblk2/1
  cfblk11/2(cfblk14) -> cfblk10/1(cfblk1)
  cfblk11/3(cfblk15) -> cfblk3/1
  cfblk4/1 -> cfblk8/1(cfblk1)
  cfblk10/1(cfblk2) -> cfblk5/1(cfblk1)
  cfblk9/1 -> cfblk10/Action
  cfblk9/2 -> cfblk11/Action
  cfblk5/1(cfblk2) -> cfblk12/1
  cfblk12/1 -> cfblk10/3(cfblk14)
  cfblk6/1(cfblk2) -> cfblk13/1
  cfblk13/1 -> cfblk11/1(cfblk1)
  cfblk3/1 -> cfblk14/1
  cfblk14/1 -> cfblk10/2(cfblk13)

== system sampleModel84/cfblk149 ==
  cfblk1 : Inport
  cfblk13 : Inport  Port=2
  Action Port : ActionPort  ActionType=else
  cfblk10 : Subsystem
  cfblk11 : Subsystem
  cfblk12 : Subsystem
  cfblk3 : Product
  cfblk4 : DotProduct  InputSameDT=on  OutDataTypeStr=Inherit: Inherit via internal rule
  cfblk5 : Abs
  cfblk6 : Reshape
  cfblk7 : ComplexToRealImag
  cfblk8 : Subsystem
  cfblk9 : Subsystem
  cfblk2 : Outport
  cfblk14 : Outport  Port=2
  cfblk15 : Outport  Port=3
  wires:
  cfblk5/1 -> cfblk14/1
  cfblk13/1 -> cfblk7/1, cfblk11/1(cfblk1)
  cfblk8/1(cfblk2) -> cfblk6/1
  cfblk11/1(cfblk2) -> cfblk2/1
  cfblk7/1 -> cfblk4/1
  cfblk12/1(cfblk2) -> cfblk8/1(cfblk1)
  cfblk1/1 -> cfblk3/1
  cfblk7/2 -> cfblk9/1(cfblk1)
  cfblk10/1(cfblk2) -> cfblk5/1
  cfblk4/1 -> cfblk12/1(cfblk1)
  cfblk3/1 -> cfblk4/2
  cfblk9/1(cfblk2) -> cfblk3/2
  cfblk6/1 -> cfblk10/1(cfblk1), cfblk15/1
